simulink model "Erreurp"  (R2014a)
settings: Solver=FixedStepDiscrete  StartTime=0.0  StopTime=2  FixedStep=Te  RelTol=1e-3
values from neighbouring files (symbols this model uses):
  DKp = Kp.den{1}    [TD6C1A2017.m]
  DP = T0d.den{1}    [TD6C1A2017.m]
  NKp = Kp.num{1}    [TD6C1A2017.m]
  NP = T0d.num{1}    [TD6C1A2017.m]
  Te = 10e-3    (= 0.01)    [TD6C1A2017.m]
settings Model: Creator=Avisse  LastModifiedBy=bavisse
settings DebuggingCC: MergeDetectMultiDrivingBlocksExec=error

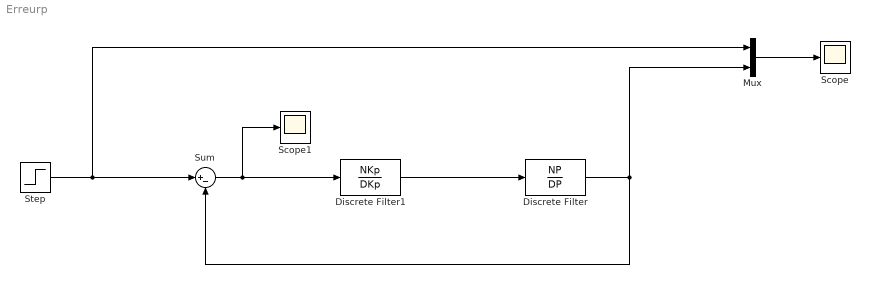
== system Erreurp ==
  Discrete Filter : DiscreteFilter  Numerator=NP  Denominator=DP  SampleTime=Te
  Discrete Filter1 : DiscreteFilter  Numerator=NKp  Denominator=DKp  SampleTime=Te
  Mux : Mux  Inputs=2
  Scope : Scope
      settings: TimeRange=2  YMin=0  YMax=6.000000000000001e+26
  Scope1 : Scope
  Step : Step  SampleTime=0
  Sum : Sum  Inputs=|+-
  wires:
  Mux/1 -> Scope/1
  Step/1 -> Mux/1, Sum/1
  Discrete Filter/1 -> Sum/2, Mux/2
  Sum/1 -> Scope1/1, Discrete Filter1/1
  Discrete Filter1/1 -> Discrete Filter/1
